simulink model "Mining_Loader_Cycle"  (R2026a)
settings: Solver=ode23t  StopTime=175  AbsTol=1e-3
PostLoadFcn:
  | sm_mining_loader_load_cycle_A
undefined symbols (not defined in the file): Maneuver
libraries: simulink x6, Maneuver_Get_Pose x2, sm_mining_loader_lib x1, Driver_Long_Lat_Stanley x1
settings Model: Creator=gabri  LastModifiedBy=smiller
settings DataIOCC: SignalLoggingName=logsout_Mining_Loader_Cycle
settings SimscapeCC: SimscapeNominalValues="[{\"value\":\"1\",\"unit\":\"A\"},{\"value\":\"1\",\"unit\":\"bar\"},{\"value\":\"1\",\"unit\":\"cm^2\"},{\"value\":\"1\",\"unit\":\"cm^3/s\"},{\"value\":\"1\",\"unit\":\"kJ/kg\"},{\"value\":\"1\",\"unit\":\"kW\"},{\"value\":\"1\",\"unit\":\"l\"},{\"value\":\"1\",\"unit\":\"N\"},{\"value\":\"1\",\"unit\":\"N*m\"},{\"value\":\"1\",\"unit\":\"V\"}]"  SimscapeLogName=simlog_Mining_Loader_Cycle  SimscapeLogLimitData=off  SimscapeLogDataHistory=5000.0
settings DiagnosticsConfigSet: SimMechanicsUnconnectedFramePorts=none  SimMechanicsUnconnectedGeometryPorts=none  SimMechanicsConflictingReferenceFrames=none
settings ExplorerConfigSet: InternalSimMechanicsExplorerSettings="<ExplorerConfiguration><canonicalview>default</canonicalview><TilePanel><TileInfo><Tiles Columns=\"2\" Count=\"2\" Height=\"611\" Rows=\"1\" Width=\"1567\"><Row Weight=\"1\"/><Column Weight=\"0.5\"/><Column Weight=\"0.5\"/><Tile Height=\"1\" Width=\"1\" X=\"0\" Y=\"0\"/><Tile Height=\"1\" Width=\"1\" X=\"1\" Y=\"0\"/></Tiles></TileInfo><SceneInfo><SceneViewer><IsThisViewStd><IsStandardView>off</IsStandardView><StandardViewName>Front</StandardViewName></IsThisViewStd><BGColor><R>1</R><G>1</G><B>1</B><A>1</A></BGColor><Camera><DoPerspective>on</DoPerspective><Position><X>1.2116701225662183</X><Y>0.99932449736717732</Y><Z>3.9888609857610082</Z></Position><Center><X>10.180869717241226</X><Y>6.0583987140410356</Y><Z>1.9990804197016925</Z></Center><Up><X>0.16524414785212499</X><Y>0.093205909739287024</Y><Z>0.98183859671042517</Z></Up><XLim>4.8906759784246461</XLim><YLim>4.8906759784246461</YLim><ViewLimDist>0.01</ViewLimDist></Camera></SceneViewer><SceneViewer><IsThisViewStd><IsStandardView>off</IsStandardView><StandardViewName>Front</StandardViewName></IsThisViewStd><BGColor><R>1</R><G>1</G><B>1</B><A>1</A></BGColor><Camera><DoPerspective>off</DoPerspective><Position><X>38.628667254344293</X><Y>-3.3655006633627913</Y><Z>803.8308353679904</Z></Position><Center><X>38.628667254344293</X><Y>-3.3655006633627913</Y><Z>1.4739994002368315</Z></Center><Up><X>-0.99996192306417131</X><Y>-0.0087265354983737543</Y><Z>0</Z></Up><XLim>36.352599481825862</XLim><YLim>36.352599481825862</YLim><ViewLimDist>0.01</ViewLimDist></Camera></SceneViewer></SceneInfo></TilePanel><MechEditorPanel><GfxPanelCameraMap><MapElement CameraMLId=\"Camera3\" GfxPanelIndex=\"0\"/></GfxPanelCameraMap><Cameras><Camera><Id>Camera1</Id><Value><Name>Track LR</Name><NativeCamera><PositionTrackingFeature>Mining_Loader.Vehicle.Camera_Frames_R.Cam_Ref_LR.R</PositionTrackingFeature><CenterTrackingFeature>Mining_Loader.Vehicle.Camera_Frames_R.Cam_Ref_Ctr.R</CenterTrackingFeature><UpVectorTrackingFeature>Mining_Loader.World_Frame.W</UpVectorTrackingFeature><CenterTrackingOrigin>on</CenterTrackingOrigin><UpVectorTrackingDirection>+Z</UpVectorTrackingDirection></NativeCamera></Value></Camera><Camera><Id>Camera2</Id><Value><Name>Track RR</Name><NativeCamera><PositionTrackingFeature>Mining_Loader.Vehicle.Camera_Frames_R.Cam_Ref_RR.R</PositionTrackingFeature><CenterTrackingFeature>Mining_Loader.Vehicle.Camera_Frames_R.Cam_Ref_Ctr.R</CenterTrackingFeature><UpVectorTrackingFeature>Mining_Loader.World_Frame.W</UpVectorTrackingFeature><CenterTrackingOrigin>on</CenterTrackingOrigin><UpVectorTrackingDirection>+Z</UpVectorTrackingDirection></NativeCamera></Value></Camera><Camera><Id>Camera3</Id><Value><Name>Track FL</Name><NativeCamera><PositionTrackingFeature>Mining_Loader.Vehicle.Camera_Frames_F.Cam_Ref_FL.R</PositionTrackingFeature><CenterTrackingFeature>Mining_Loader.Vehicle.Camera_Frames_F.Cam_Ref_Ctr.R</CenterTrackingFeature><UpVectorTrackingFeature>Mining_Loader.World_Frame.W</UpVectorTrackingFeature><CenterTrackingOrigin>on</CenterTrackingOrigin><UpVectorTrackingDirection>+Z</UpVectorTrackingDirection></NativeCamera></Value></Camera><Camera><Id>Camera4</Id><Value><Name>Track FR</Name><NativeCamera><PositionTrackingFeature>Mining_Loader.Vehicle.Camera_Frames_F.Cam_Ref_FR.R</PositionTrackingFeature><CenterTrackingFeature>Mining_Loader.Vehicle.Camera_Frames_F.Cam_Ref_Ctr.R</CenterTrackingFeature><UpVectorTrackingFeature>Mining_Loader.World_Frame.W</UpVectorTrackingFeature><CenterTrackingOrigin>on</CenterTrackingOrigin><UpVectorTrackingDirection>+Z</UpVectorTrackingDirection></NativeCamera></Value></Camera><Camera><Id>Camera5</Id><Value><Name>Track Frame Right</Name><NativeCamera><PositionTrackingFeature>Mining_Loader.Vehicle.Camera_Frames_F.Cam_Ref_Right.R</PositionTrackingFeature><CenterTrackingFeature>Mining_Loader.Vehicle.Camera_Frames_F.Cam_Ref_Right.R</CenterTrackingFeature><UpVectorTrackingFeature>Mining_Loader.World_Frame.W</UpVectorTrackingFeature><CenterTrackingOrigin>off</CenterTrackingOrigin><CenterTrackingDirection>-Y</CenterTrackingDirection><UpVectorTrackingDirection>+Z</UpVectorTrackingDirection></NativeCamera></Value></Camera><Camera><Id>Camera6</Id><Value><Name>Track Frame Left</Name><NativeCamera><PositionTrackingFeature>Mining_Loader.Vehicle.Camera_Frames_F.Cam_Ref_Left.R</PositionTrackingFeature><CenterTrackingFeature>Mining_Loader.Vehicle.Camera_Frames_F.Cam_Ref_Left.R</CenterTrackingFeature><UpVectorTrackingFeature>Mining_Loader.World_Frame.W</UpVectorTrackingFeature><CenterTrackingOrigin>off</CenterTrackingOrigin><CenterTrackingDirection>+Y</CenterTrackingDirection><UpVectorTrackingDirection>+Z</UpVectorTrackingDirection></NativeCamera></Value></Camera><Camera><Id>Camera7</Id><Value><Name>Track Frame Top Down</Name><NativeCamera><PositionTrackingFeature>Mining_Loader.Vehicle.Camera_Frames_F.Cam_Ref_Top_Down.R</PositionTrackingFeature><CenterTrackingFeature>Mining_Loader.Vehicle.Camera_Frames_F.Cam_Ref_Top_Down.R</CenterTrackingFeature><UpVectorTrackingFeature>Mining_Loader.Vehicle.Camera_Frames_F.Cam_Ref_Top_Down.R</UpVectorTrackingFeature><CenterTrackingOrigin>off</CenterTrackingOrigin><CenterTrackingDirection>-Z</CenterTrackingDirection><UpVectorTrackingDirection>+Y</UpVectorTrackingDirection></NativeCamera></Value></Camera><Camera><Id>Camera8</Id><Value><Name>Track Frame Rear Fwd</Name><NativeCamera><PositionTrackingFeature>Mining_Loader.Vehicle.Camera_Frames_F.Cam_Ref_Top_Rear_Fwd.R</PositionTrackingFeature><CenterTrackingFeature>Mining_Loader.Vehicle.Camera_Frames_F.Cam_Ref_Top_Rear_Fwd.R</CenterTrackingFeature><UpVectorTrackingFeature>Mining_Loader.World_Frame.W</UpVectorTrackingFeature><CenterTrackingOrigin>off</CenterTrackingOrigin><CenterTrackingDirection>+X</CenterTrackingDirection><UpVectorTrackingDirection>+Z</UpVectorTrackingDirection></NativeCamera></Value></Camera><Camera><Id>Camera9</Id><Value><Name>Track Chassis Right</Name><NativeCamera><PositionTrackingFeature>Mining_Loader.Vehicle.Camera_Frames_R.Cam_Ref_Right.R</PositionTrackingFeature><CenterTrackingFeature>Mining_Loader.Vehicle.Camera_Frames_R.Cam_Ref_Right.R</CenterTrackingFeature><UpVectorTrackingFeature>Mining_Loader.World_Frame.W</UpVectorTrackingFeature><CenterTrackingOrigin>off</CenterTrackingOrigin><CenterTrackingDirection>-Y</CenterTrackingDirection><UpVectorTrackingDirection>+Z</UpVectorTrackingDirection></NativeCamera></Value></Camera><Camera><Id>Camera10</Id><Value><Name>Track Chassis Left</Name><NativeCamera><PositionTrackingFeature>Mining_Loader.Vehicle.Camera_Frames_F.Cam_Ref_Left.R</PositionTrackingFeature><CenterTrackingFeature>Mining_Loader.Vehicle.Camera_Frames_F.Cam_Ref_Left.R</CenterTrackingFeature><UpVectorTrackingFeature>Mining_Loader.World_Frame.W</UpVectorTrackingFeature><CenterTrackingOrigin>off</CenterTrackingOrigin><CenterTrackingDirection>+Y</CenterTrackingDirection><UpVectorTrackingDirection>+Z</UpVectorTrackingDirection></NativeCamera></Value></Camera><Camera><Id>Camera11</Id><Value><Name>Track Chassis Top Down</Name><NativeCamera><PositionTrackingFeature>Mining_Loader.Vehicle.Camera_Frames_R.Cam_Ref_Top_Down.R</PositionTrackingFeature><CenterTrackingFeature>Mining_Loader.Vehicle.Camera_Frames_R.Cam_Ref_Top_Down.R</CenterTrackingFeature><UpVectorTrackingFeature>Mining_Loader.Vehicle.Camera_Frames_R.Cam_Ref_Top_Down.R</UpVectorTrackingFeature><CenterTrackingOrigin>off</CenterTrackingOrigin><CenterTrackingDirection>-Z</CenterTrackingDirection><UpVectorTrackingDirection>+Y</UpVectorTrackingDirection></NativeCamera></Value></Camera><Camera><Id>Camera12</Id><Value><Name>Track Chassis Rear Fwd</Name><NativeCamera><PositionTrackingFeature>Mining_Loader.Vehicle.Camera_Frames_R.Cam_Ref_Top_Rear_Fwd.R</PositionTrackingFeature><CenterTrackingFeature>Mining_Loader.Vehicle.Camera_Frames_R.Cam_Ref_Top_Rear_Fwd.R</CenterTrackingFeature><UpVectorTrackingFeature>Mining_Loader.World_Frame.W</UpVectorTrackingFeature><CenterTrackingOrigin>off</CenterTrackingOrigin><CenterTrackingDirection>+X</CenterTrackingDirection><UpVectorTrackingDirection>+Z</UpVectorTrackingDirection></NativeCamera></Value></Camera></Cameras><VideoCreator><IncludeTiles>All</IncludeTiles><IncludeTime>on</IncludeTime><IncludeWorldFrame>off</IncludeWorldFrame><PlaybackSpeedRatio>1</PlaybackSpeedRatio><FrameRate>30</FrameRate><FrameSize>auto</FrameSize><VideoFormat>UncompressedAVI</VideoFormat></VideoCreator></MechEditorPanel><PlaybackSettings><PlaybackSpeedFactor>8</PlaybackSpeedFactor></PlaybackSettings></ExplorerConfiguration>"

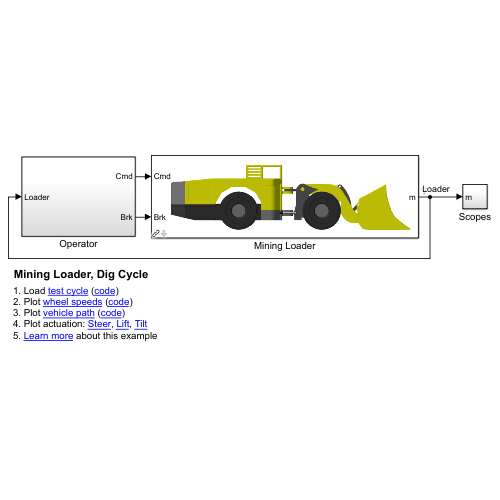
[thumbnail: Simulink's stored preview of the top-level diagram]
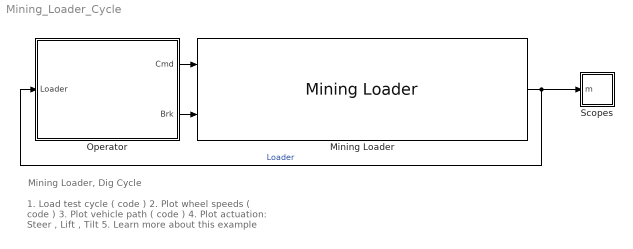
== system Mining_Loader_Cycle ==
  note: 1. Load test cycle ( code )
      | 2. Plot wheel speeds ( code )
      | 3. Plot vehicle path ( code )
      | 4. Plot actuation: Steer , Lift , Tilt
      | 5. Learn more about this example
  note: Mining Loader, Dig Cycle
  Mining Loader : sm_mining_loader_lib/Mining Loader  popup_steer_actuation=Hinge Motion  popup_lift_actuation=Hinge Motion  popup_tilt_actuation=Hinge Motion  popup_scene=Grid  popup_sensor=Estimate
  Operator : Subsystem
  Scopes : Subsystem
  wires:
  Mining Loader/1 -> Operator/1(Loader), Scopes/1(m)  "Loader"
  Operator/1(Cmd) -> Mining Loader/1
  Operator/2(Brk) -> Mining Loader/2

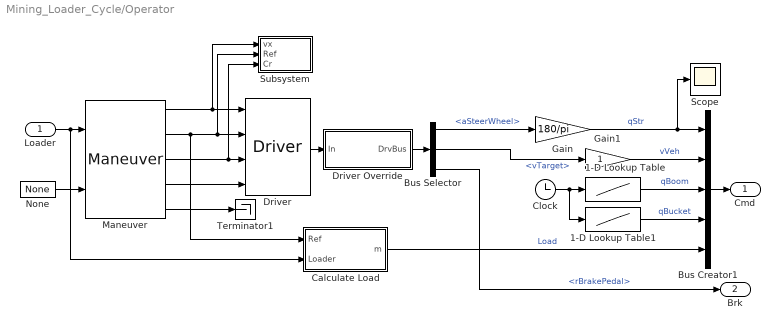
== system Mining_Loader_Cycle/Operator ==
  Loader : Inport
  1-D Lookup Table : Lookup_n-D  NumberOfTableDimensions=1  BreakpointsForDimension1=Maneuver.Impl.Boom.t.Value  Table=Maneuver.Impl.Boom.q.Value  InternalRulePriority=Speed  RndMeth=Simplest
  1-D Lookup Table1 : Lookup_n-D  NumberOfTableDimensions=1  BreakpointsForDimension1=Maneuver.Impl.Bucket.t.Value  Table=Maneuver.Impl.Bucket.q.Value  InternalRulePriority=Speed  RndMeth=Simplest
  Bus Creator1 : BusCreator  Inputs=5
  Bus Selector : BusSelector  OutputSignals=aSteerWheel,signal1.vTarget,rBrakePedal
  Calculate Load : Subsystem  mask{upTilt=-45, downTilt=45, xPile=74.25, dPile=3, loadMax=10000}
      mask prompts: upTilt "Angle Bucket Tilt Up (deg)"; downTilt "Angle Bucket Tilt Down (deg)"; xPile "Distance to start of pile (m)"; dPile "Depth of pile (m)"; loadMax "Max Load (kg)"
  Clock : Clock
  Driver : Driver_Long_Lat_Stanley/Driver  Driver=Driver
  Driver Override : Subsystem  Variant=on  VariantControlMode=label  VariantControl=Choice  LabelModeActiveChoice=Override  mask(Override Driver Commands){popup_driver_override=Override}
      mask prompts: popup_driver_override "Driver Override"
      mask help: Override closed-loop driver commands with open-loop inputs. Can be applied to steering wheel, accelerator pedal. or brake pedal.
      mask init:
      | curblk = gcb;
      | 
      | set_param(curblk,'LabelModeActiveChoice',get_param(curblk,'popup_driver_override'));
      mask TypeOptions popup_driver_override: None | Override
  Gain : Gain  Gain=180/pi
  Gain1 : Gain
  Maneuver : Maneuver_Get_Pose/Maneuver  Maneuver=Maneuver  popup_window=No
  None : Maneuver_Get_Pose/None  SystemSampleTime=-1  VariantControl=None  VariantActivationTime=update diagram  EmptyChoice=off  PassThrough=off  PassThroughVariantControl=(default)  EmptyChoiceVariantControl=(default)  AllowFlexibleInterface=on  Latency=0  AutoFrameSizeCalculation=off
  Scope : Scope
      settings: ActiveDisplayYMinimum=-70.82509949755412  ActiveDisplayYMaximum=68.336364755935136  DataLoggingVariableName=ScopeData6
  Subsystem : Subsystem
  Terminator1 : Terminator
  Cmd : Outport
  Brk : Outport  Port=2
  wires:
  Maneuver/1 -> Subsystem/1(vx), Driver/1
  None/1 -> Maneuver/2
  Maneuver/5 -> Terminator1/1
  Maneuver/2 -> Calculate Load/1(Ref), Subsystem/2(Ref), Driver/2
  Maneuver/4 -> Driver/4
  Loader/1 -> Calculate Load/2(Loader), Maneuver/1
  1-D Lookup Table1/1 -> Bus Creator1/4  "qBucket"
  Clock/1 -> 1-D Lookup Table1/1, 1-D Lookup Table/1
  Bus Selector/2 -> Gain1/1  "<vTarget>"
  Driver Override/1(DrvBus) -> Bus Selector/1
  Gain/1 -> Scope/1, Bus Creator1/1  "qStr"
  Gain1/1 -> Bus Creator1/2  "vVeh"
  Bus Selector/1 -> Gain/1  "<aSteerWheel>"
  Bus Selector/3 -> Brk/1  "<rBrakePedal>"
  Bus Creator1/1 -> Cmd/1
  1-D Lookup Table/1 -> Bus Creator1/3  "qBoom"
  Driver/1 -> Driver Override/1(In)
  Maneuver/3 -> Subsystem/3(Cr), Driver/3
  Calculate Load/1(m) -> Bus Creator1/5  "Load"

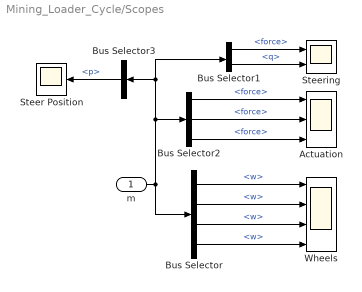
== system Mining_Loader_Cycle/Scopes ==
  m : Inport
  Actuation : Scope  NumInputPorts=3
      settings: ActiveDisplayYMinimum=-159687.98470952915  ActiveDisplayYMaximum=143959.05671016159  DataLoggingVariableName=ScopeData3
  Bus Selector : BusSelector  OutputSignals=Vehicle.Frame.WhlFL.w,Vehicle.Frame.WhlFR.w,Vehicle.Chassis.WhlRL.w,Vehicle.Chassis.WhlRR.w
  Bus Selector1 : BusSelector  OutputSignals=Vehicle.Steer.L.force,Vehicle.Steer.H.q
  Bus Selector2 : BusSelector  OutputSignals=Vehicle.Steer.L.force,Vehicle.Lift.L.force,Vehicle.Tilt.A.force
  Bus Selector3 : BusSelector  OutputSignals=Vehicle.Steer.L.p
  Steer Position : Scope
      settings: ActiveDisplayYMinimum=0.3695595859326416  ActiveDisplayYMaximum=0.37940534904193796  DataLoggingVariableName=ScopeData5
  Steering : Scope  NumInputPorts=2
      settings: ActiveDisplayYMinimum=-11000  ActiveDisplayYMaximum=-9000  DataLoggingVariableName=ScopeData2
  Wheels : Scope  NumInputPorts=4
      settings: ActiveDisplayYMinimum=-3.3536402711146023  ActiveDisplayYMaximum=3.6534134238864517
  wires:
  m/1 -> Bus Selector1/1, Bus Selector3/1, Bus Selector2/1, Bus Selector/1
  Bus Selector/2 -> Wheels/2  "<w>"
  Bus Selector/1 -> Wheels/1  "<w>"
  Bus Selector/3 -> Wheels/3  "<w>"
  Bus Selector/4 -> Wheels/4  "<w>"
  Bus Selector1/1 -> Steering/1  "<force>"
  Bus Selector1/2 -> Steering/2  "<q>"
  Bus Selector2/2 -> Actuation/2  "<force>"
  Bus Selector2/3 -> Actuation/3  "<force>"
  Bus Selector3/1 -> Steer Position/1  "<p>"
  Bus Selector2/1 -> Actuation/1  "<force>"

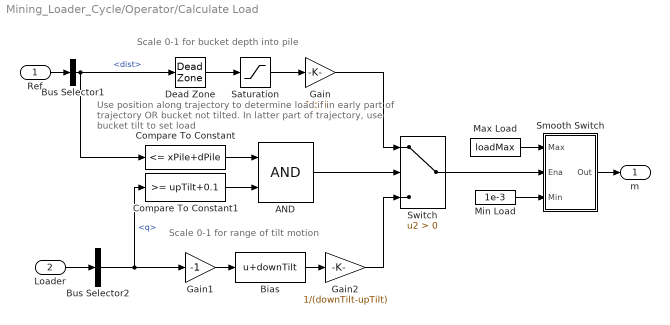
== system Mining_Loader_Cycle/Operator/Calculate Load ==
  note: Scale 0-1 for bucket depth into pile
  note: Scale 0-1 for range of tilt motion
  note: Use position along trajectory to determine load
      | if in early part of trajectory OR bucket not tilted.
      | In latter part of trajectory, use bucket tilt to set load
  Ref : Inport
  Loader : Inport  Port=2
  AND : Logic  IconShape=distinctive  AllPortsSameDT=off  OutDataTypeStr=boolean
  Bias : Bias  Bias=downTilt  SaturateOnIntegerOverflow=off
  Bus Selector1 : BusSelector  OutputSignals=dist
  Bus Selector2 : BusSelector  OutputSignals=Vehicle.Tilt.H.q
  Compare To Constant : simulink/Logic and Bit Operations/Compare To Constant  relop=<=  const=xPile+dPile  OutDataTypeStr=boolean
  Compare To Constant1 : simulink/Logic and Bit Operations/Compare To Constant  relop=>=  const=upTilt+0.1  OutDataTypeStr=boolean
  Dead Zone : DeadZone  LowerValue=-xPile  UpperValue=xPile  ZeroCross=off
  Gain : Gain  Gain=1/dPile
  Gain1 : Gain  Gain=-1
  Gain2 : Gain  Gain=1/(downTilt-upTilt)
  Max Load : Constant  Value=loadMax
  Min Load : Constant  Value=1e-3
  Saturation : Saturate  UpperLimit=dPile  LowerLimit=0
  Smooth Switch : Subsystem
  Switch : Switch  Criteria=u2 > Threshold  SaturateOnIntegerOverflow=off  InputSameDT=off
  m : Outport
  wires:
  Bus Selector1/1 -> Dead Zone/1, Compare To Constant/1  "<dist>"
  Bus Selector2/1 -> Gain1/1, Compare To Constant1/1  "<q>"
  Smooth Switch/1(Out) -> m/1
  Ref/1 -> Bus Selector1/1
  Loader/1 -> Bus Selector2/1
  Min Load/1 -> Smooth Switch/3(Min)
  Compare To Constant/1 -> AND/1
  Dead Zone/1 -> Saturation/1
  Saturation/1 -> Gain/1
  Gain/1 -> Switch/1
  AND/1 -> Switch/2
  Compare To Constant1/1 -> AND/2
  Gain1/1 -> Bias/1
  Bias/1 -> Gain2/1
  Gain2/1 -> Switch/3
  Switch/1 -> Smooth Switch/2(Ena)
  Max Load/1 -> Smooth Switch/1(Max)

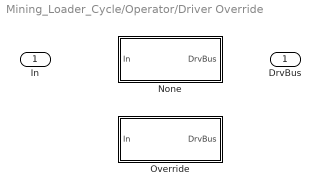
== system Mining_Loader_Cycle/Operator/Driver Override ==
  In : Inport
  None : Subsystem  VariantControl=None
  Override : Subsystem  VariantControl=Override
  DrvBus : Outport

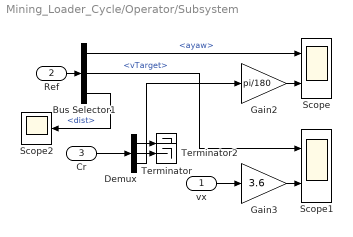
== system Mining_Loader_Cycle/Operator/Subsystem ==
  vx : Inport
  Ref : Inport  Port=2
  Cr : Inport  Port=3
  Bus Selector1 : BusSelector  OutputSignals=ayaw,vTarget,dist
  Demux : Demux  Outputs=3
  Gain2 : Gain  Gain=pi/180
  Gain3 : Gain  Gain=3.6
  Scope : Scope  NumInputPorts=2
      settings: ActiveDisplayYMinimum=-12.759963955341339  ActiveDisplayYMaximum=4.9084322768043629
  Scope1 : Scope  NumInputPorts=2
      settings: ActiveDisplayYMinimum=-0.88489867104719  ActiveDisplayYMaximum=5.6538776301163542  DataLoggingVariableName=ScopeData4
  Scope2 : Scope
      settings: ActiveDisplayYMinimum=77.173432371850652  ActiveDisplayYMaximum=77.26142474505312  DataLoggingVariableName=ScopeData7
  Terminator : Terminator
  Terminator2 : Terminator
  wires:
  vx/1 -> Gain3/1
  Cr/1 -> Demux/1
  Ref/1 -> Bus Selector1/1
  Gain3/1 -> Scope1/2
  Demux/1 -> Terminator/1
  Demux/3 -> Gain2/1
  Gain2/1 -> Scope/2
  Demux/2 -> Terminator2/1
  Bus Selector1/1 -> Scope/1  "<ayaw>"
  Bus Selector1/2 -> Scope1/1  "<vTarget>"
  Bus Selector1/3 -> Scope2/1  "<dist>"

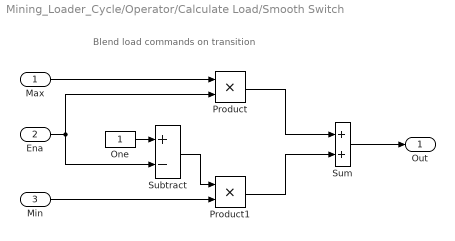
== system Mining_Loader_Cycle/Operator/Calculate Load/Smooth Switch ==
  note: Blend load commands on transition
  Max : Inport
  Ena : Inport  Port=2
  Min : Inport  Port=3
  One : Constant  OutDataTypeStr=Inherit: Inherit via back propagation
  Product : Product
  Product1 : Product
  Subtract : Sum  Inputs=+-
  Sum : Sum
  Out : Outport
  wires:
  Max/1 -> Product/1
  Ena/1 -> Product/2, Subtract/2
  One/1 -> Subtract/1
  Subtract/1 -> Product1/1
  Min/1 -> Product1/2
  Sum/1 -> Out/1
  Product/1 -> Sum/1
  Product1/1 -> Sum/2

== system Mining_Loader_Cycle/Operator/Driver Override/None ==
  In : Inport
  DrvBus : Outport
  wires:
  In/1 -> DrvBus/1

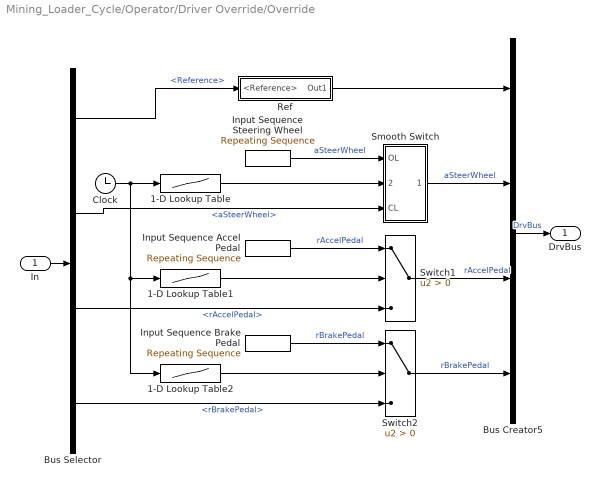
== system Mining_Loader_Cycle/Operator/Driver Override/Override ==
  In : Inport
  1-D Lookup Table : Lookup_n-D  NumberOfTableDimensions=1  BreakpointsForDimension1=Maneuver.Override.aSteer.t.Value  Table=Maneuver.Override.aSteer.On.Value  InternalRulePriority=Speed  RndMeth=Simplest
  1-D Lookup Table1 : Lookup_n-D  NumberOfTableDimensions=1  BreakpointsForDimension1=Maneuver.Override.Accel.t.Value  Table=Maneuver.Override.Accel.On.Value  InternalRulePriority=Speed  RndMeth=Simplest
  1-D Lookup Table2 : Lookup_n-D  NumberOfTableDimensions=1  BreakpointsForDimension1=Maneuver.Override.Brake.t.Value  Table=Maneuver.Override.Brake.On.Value  InternalRulePriority=Speed  RndMeth=Simplest
  Bus Creator5 : BusCreator  Inputs=4
  Bus Selector : BusSelector  OutputSignals=Reference,aSteerWheel,rAccelPedal,rBrakePedal
  Clock : Clock
  Input Sequence Accel Pedal : simulink/Sources/Repeating Sequence  rep_seq_t=Maneuver.Accel.t.Value  rep_seq_y=Maneuver.Accel.rPedal.Value
  Input Sequence Brake Pedal : simulink/Sources/Repeating Sequence  rep_seq_t=Maneuver.Brake.t.Value  rep_seq_y=Maneuver.Brake.rPedal.Value
  Input Sequence Steering Wheel : simulink/Sources/Repeating Sequence  rep_seq_t=Maneuver.Steer.t.Value  rep_seq_y=Maneuver.Steer.aWheel.Value
  Ref : Subsystem
  Smooth Switch : Subsystem
  Switch1 : Switch  Criteria=u2 > Threshold  SaturateOnIntegerOverflow=off  InputSameDT=off
  Switch2 : Switch  Criteria=u2 > Threshold  SaturateOnIntegerOverflow=off  InputSameDT=off
  DrvBus : Outport
  wires:
  Input Sequence Brake Pedal/1 -> Switch2/1  "rBrakePedal"
  Input Sequence Accel Pedal/1 -> Switch1/1  "rAccelPedal"
  Input Sequence Steering Wheel/1 -> Smooth Switch/1(OL)  "aSteerWheel"
  Switch2/1 -> Bus Creator5/4  "rBrakePedal"
  1-D Lookup Table/1 -> Smooth Switch/2(Ena)
  Clock/1 -> 1-D Lookup Table/1, 1-D Lookup Table2/1, 1-D Lookup Table1/1
  Bus Selector/4 -> Switch2/3  "<rBrakePedal>"
  Switch1/1 -> Bus Creator5/3  "rAccelPedal"
  Bus Selector/3 -> Switch1/3  "<rAccelPedal>"
  Smooth Switch/1(Out) -> Bus Creator5/2  "aSteerWheel"
  Bus Selector/2 -> Smooth Switch/3(CL)  "<aSteerWheel>"
  Bus Creator5/1 -> DrvBus/1  "DrvBus"
  In/1 -> Bus Selector/1
  1-D Lookup Table1/1 -> Switch1/2
  1-D Lookup Table2/1 -> Switch2/2
  Bus Selector/1 -> Ref/1(<Reference>)  "<Reference>"
  Ref/1(Out1) -> Bus Creator5/1

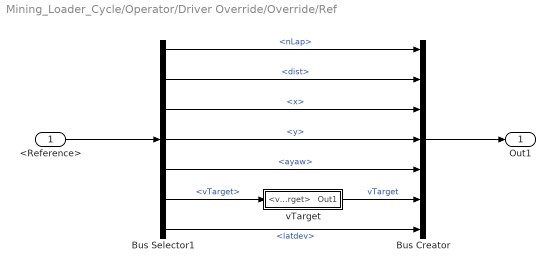
== system Mining_Loader_Cycle/Operator/Driver Override/Override/Ref ==
  <Reference> : Inport
  Bus Creator : BusCreator  Inputs=7
  Bus Selector1 : BusSelector  OutputSignals=nLap,dist,x,y,ayaw,vTarget,latdev
  vTarget : Subsystem
  Out1 : Outport
  wires:
  Bus Selector1/3 -> Bus Creator/3  "<x>"
  Bus Selector1/2 -> Bus Creator/2  "<dist>"
  Bus Selector1/1 -> Bus Creator/1  "<nLap>"
  Bus Selector1/4 -> Bus Creator/4  "<y>"
  vTarget/1(Out1) -> Bus Creator/6  "vTarget"
  Bus Selector1/6 -> vTarget/1(<vTarget>)  "<vTarget>"
  Bus Selector1/7 -> Bus Creator/7  "<latdev>"
  Bus Selector1/5 -> Bus Creator/5  "<ayaw>"
  <Reference>/1 -> Bus Selector1/1
  Bus Creator/1 -> Out1/1

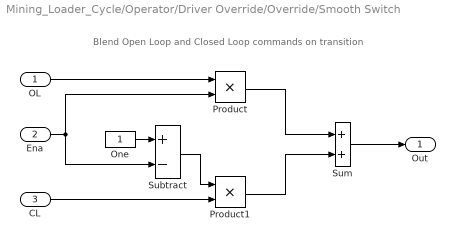
== system Mining_Loader_Cycle/Operator/Driver Override/Override/Smooth Switch ==
  note: Blend Open Loop and
      | Closed Loop commands on transition
  OL : Inport
  Ena : Inport  Port=2
  CL : Inport  Port=3
  One : Constant  OutDataTypeStr=Inherit: Inherit via back propagation
  Product : Product
  Product1 : Product
  Subtract : Sum  Inputs=+-
  Sum : Sum
  Out : Outport
  wires:
  OL/1 -> Product/1
  Ena/1 -> Product/2, Subtract/2
  One/1 -> Subtract/1
  Subtract/1 -> Product1/1
  CL/1 -> Product1/2
  Sum/1 -> Out/1
  Product/1 -> Sum/1
  Product1/1 -> Sum/2

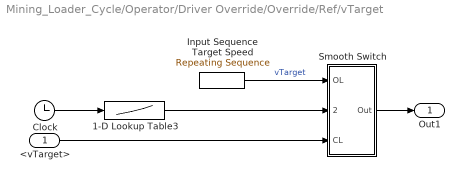
== system Mining_Loader_Cycle/Operator/Driver Override/Override/Ref/vTarget ==
  <vTarget> : Inport
  1-D Lookup Table3 : Lookup_n-D  NumberOfTableDimensions=1  BreakpointsForDimension1=Maneuver.Override.vTarget.t.Value  Table=Maneuver.Override.vTarget.On.Value  InternalRulePriority=Speed  RndMeth=Simplest
  Clock : Clock
  Input Sequence Target Speed : simulink/Sources/Repeating Sequence  rep_seq_t=Maneuver.vTarget.t.Value  rep_seq_y=Maneuver.vTarget.kph.Value
  Smooth Switch : Subsystem
  Out1 : Outport
  wires:
  Smooth Switch/1(Out) -> Out1/1
  <vTarget>/1 -> Smooth Switch/3(CL)
  Clock/1 -> 1-D Lookup Table3/1
  Input Sequence Target Speed/1 -> Smooth Switch/1(OL)  "vTarget"
  1-D Lookup Table3/1 -> Smooth Switch/2(Ena)

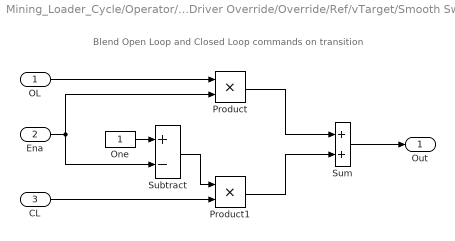
== system Mining_Loader_Cycle/Operator/Driver Override/Override/Ref/vTarget/Smooth Switch ==
  note: Blend Open Loop and
      | Closed Loop commands on transition
  OL : Inport
  Ena : Inport  Port=2
  CL : Inport  Port=3
  One : Constant  OutDataTypeStr=Inherit: Inherit via back propagation
  Product : Product
  Product1 : Product
  Subtract : Sum  Inputs=+-
  Sum : Sum
  Out : Outport
  wires:
  OL/1 -> Product/1
  Ena/1 -> Product/2, Subtract/2
  One/1 -> Subtract/1
  Subtract/1 -> Product1/1
  CL/1 -> Product1/2
  Sum/1 -> Out/1
  Product/1 -> Sum/1
  Product1/1 -> Sum/2
